simulink model "pe_estim_int_dump"  (Simulink 8.7)
settings: Solver=FixedStepDiscrete  SolverMode=SingleTasking  StartTime=0.0  StopTime=5000e-3  FixedStep=1/100000  RelTol=1e-3
libraries: commchan3 x1, commsink2 x1, commfilt2 x1, dspsrcs4 x1, commutil2 x1
settings Model: Creator=amoura  LastModifiedBy=Artur Moura
settings DataIOCC: LimitDataPoints=off  SignalLoggingSaveFormat=ModelDataLogs  SignalLoggingName=sigsOut
settings OptimizationCC: BooleanDataType=off  ExpressionDepthLimit=2147483647  InitFltsAndDblsToZero=on
settings DebuggingCC: SaveWithParameterizedLinksMsg=none  SignalResolutionControl=TryResolveAllWithWarning  MultiTaskDSMMsg=warning  MultiTaskCondExecSysMsg=none  FcnCallInpInsideContextMsg=UseLocalSettings  StateNameClashWarn=warning
settings HardwareCC: TargetUnknown=on
settings RTWCC: TemplateMakefile=grt_unix.tmf
settings GRTTargetCC: TargetFcnLib=ansi_tfl_tmw.mat  ModelReferenceCompliant=off  CombineOutputUpdateFcns=off  MatFileLogging=off  GRTInterface=on

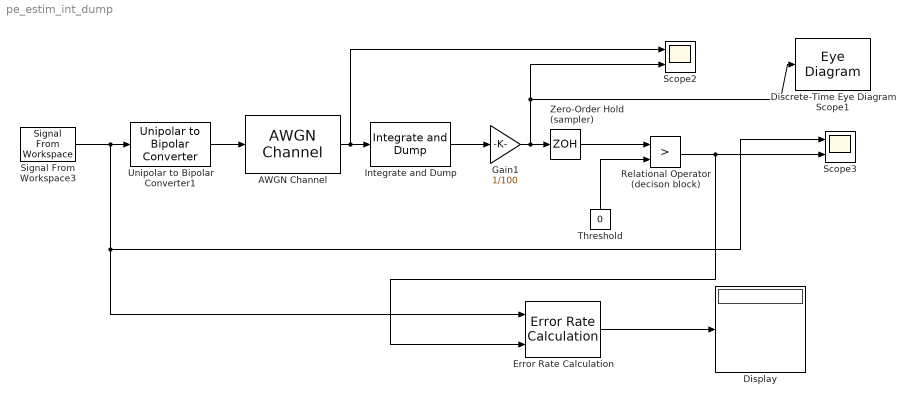
== system pe_estim_int_dump ==
  AWGN Channel : commchan3/AWGN Channel  InputProcessing=Columns as channels (frame based)  seed=79  noiseMode=Variance from mask  EbNodB=10  EsNodB=10  SNRdB=10  bitsPerSym=1  Ps=1  Tsym=1  variance=20
  Discrete-Time Eye Diagram Scope1 : EyeDiagram  Tag=EyeDiagram
  Display : Display
  Error Rate Calculation : commsink2/Error Rate Calculation  N=1  st_delay=0  cp_mode=Entire frame  subframe=[]  PMode=Port  WsName=ErrorVec  RsMode2=off  stop=off  numErr=100  maxBits=1e6
  Gain1 : Gain  Gain=1/100  RndMeth=Nearest  SampleTime=1/100000  SaturateOnIntegerOverflow=on  OutDataTypeStr=Inherit: Same as input  ParamDataTypeStr=Inherit: Same as input
  Integrate and Dump : commfilt2/Integrate and Dump  obssamples=100  offsetsamples=1  nodump=on  roundingMode=Floor  overflowMode=off  outputDataTypeStr=Inherit: Same as accumulator  outputLastDataTypeStr=Inherit: Same as accumulator
  Relational Operator (decison block) : RelationalOperator  Operator=>  InputSameDT=on
  Scope2 : Scope  NumInputPorts=2
  Scope3 : Scope  NumInputPorts=2
  Signal From Workspace3 : dspsrcs4/Signal From Workspace  X=randi([0 1],10000,1)  Ts=1/1000  nsamps=1  OutputAfterFinalValue=Cyclic repetition  ignoreOrWarnInputAndFrameLengths=off  OutputFrames=on
  Threshold : Constant  Value=0
  Unipolar to Bipolar Converter1 : commutil2/Unipolar to Bipolar Converter  M=2  polarity=Positive  dataType=Same as input
  Zero-Order Hold (sampler) : ZeroOrderHold  SampleTime=1/1000
  wires:
  Integrate and Dump/1 -> Gain1/1
  Signal From Workspace3/1 -> Error Rate Calculation/1, Scope3/1, Unipolar to Bipolar Converter1/1
  Unipolar to Bipolar Converter1/1 -> AWGN Channel/1
  AWGN Channel/1 -> Integrate and Dump/1, Scope2/1
  Error Rate Calculation/1 -> Display/1
  Zero-Order Hold (sampler)/1 -> Relational Operator (decison block)/1
  Relational Operator (decison block)/1 -> Error Rate Calculation/2, Scope3/2
  Threshold/1 -> Relational Operator (decison block)/2
  Gain1/1 -> Zero-Order Hold (sampler)/1, Discrete-Time Eye Diagram Scope1/1, Scope2/2
